simulink library "relay_tripOutMng_lib"  (Simulink 8.1)
settings: Solver=ode45  StartTime=0.0  StopTime=10.0  RelTol=1e-3
settings Model: Creator=RE25624  LastModifiedBy=RE25624

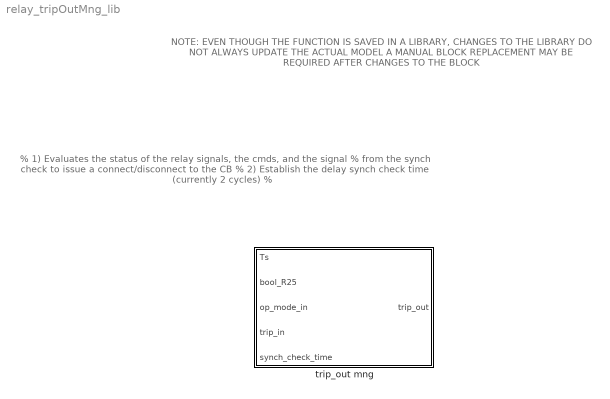
== system relay_tripOutMng_lib ==
  note: NOTE:  EVEN THOUGH THE FUNCTION IS SAVED IN A LIBRARY, CHANGES TO THE LIBRARY DO NOT ALWAYS UPDATE THE ACTUAL MODEL
      |
      | A MANUAL BLOCK REPLACEMENT MAY BE REQUIRED AFTER CHANGES TO THE BLOCK
  note: % 1) Evaluates the status of the relay signals, the cmds, and the signal
      | % from the synch check to issue a connect/disconnect to the CB
      | % 2) Establish the delay synch check time (currently 2 cycles)
      | %
  trip_out mng : MATLAB Function  TreatAsAtomicUnit=on

== matlab function trip_out mng ==
  data: Ts input double; bool_R25 input double; op_mode_in input double; trip_out output double; trip_in input double; synch_check_time input double
% CREATED BY: REYNALDO SALCEDO
% LAST CHANGE BY : REYNALDO SALCEDO
% GROUP: 73
% DATE MODIFIED  : 04/19/2016
%

% 1) Evaluates the status of the relay signals, the cmds, and the signal 
% from the synch check to issue a connect/disconnect to the CB
% 2) Establish the delay synch check time (currently 2 cycles)
%

function trip_out = opModeChk(Ts, bool_R25, op_mode_in, trip_in, synch_check_time)
%#codegen

persistent n25 prev_mode prev_trip_in
if isempty(prev_mode)
    n25 = 0; % time counter
    prev_mode = 0; % initially operating on logic
    prev_trip_in = 1; % initially close
end

trip_out = trip_in * bool_R25;

% the R25 logic will be active if the breaker has been opened, and a
% forced-to-close command is applied
if (prev_mode==2 || prev_trip_in==0) && (op_mode_in==1 || op_mode_in==0) && trip_in==1
    
    % time accumulation
    n25 = n25 * bool_R25;
    n25 = n25 + bool_R25 * Ts;
    if n25 > synch_check_time
        trip_out = 1;
        % reset history values
        prev_mode = op_mode_in;
        prev_trip_in = trip_in;
    else
        prev_mode = 2;
        prev_trip_in = 0;
        trip_out = 0;
    end
    
elseif op_mode_in==2
    prev_mode = 2;
    prev_trip_in = 0;
    trip_out = 0;
    n25 = 0;
else
    n25 = 0;
end
